simulink model "SelfAndRegularCheckouts"  (R2020a)
settings: Solver=VariableStepAuto  StartTime=0.0  StopTime=10.0  RelTol=1e-3
undefined symbols (not defined in the file): m, n
libraries: dspstat3 x1
settings Model: Creator=jggam  LastModifiedBy=jggam

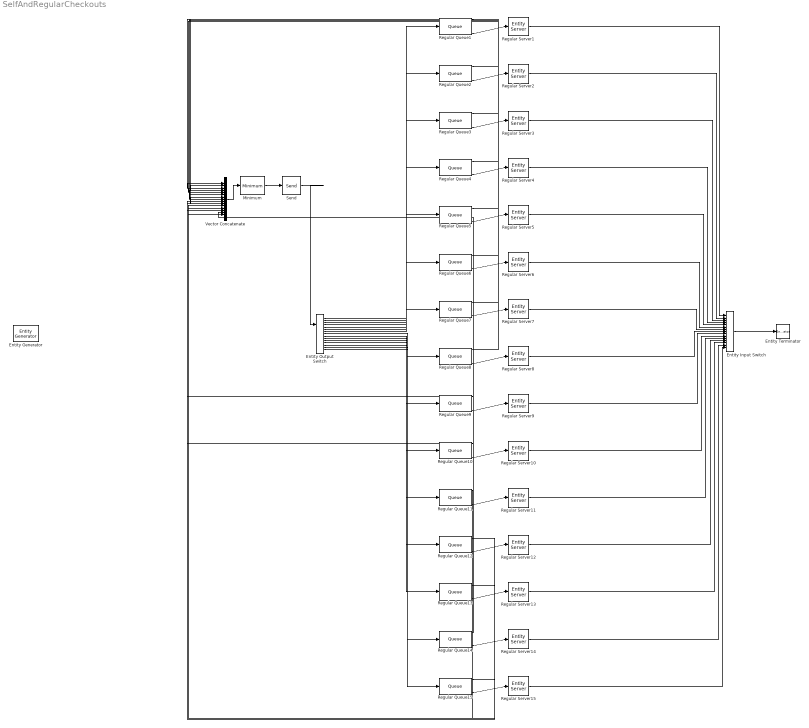
== system SelfAndRegularCheckouts ==
  Entity Input Switch : EntityInputSwitch  InputPortMessageModes=m,m,m,m,m,m,m,m,m,m,m,m,m,m,m  OutputPortMessageModes=m  NumberInputPorts=15
      settings: InputPortMap=u1,u2,u3,u4,u5,u6,u7,u8,u9,u10,u11,u12,u13,u14,u15
  Entity Output Switch : EntityOutputSwitch  InputPortMessageModes=m,m  OutputPortMessageModes=m,m,m,m,m,m,m,m,m,m,m,m,m,m,m  NumberOutputPorts=15  SwitchingCriterion=From control port  SwitchAttributeName=Attribute1
      settings: InputPortMap=u0,u1  OutputPortMap=o0,o1,o2,o3,o4,o5,o6,o7,o8,o9,o10,o11,o12,o13,o14
  Entity Generator : EntityGenerator  OutputPortMessageModes=n,m  TimeSource=MATLAB action  Period=0.5  IntergenerationTimeAction=dt = arrivalTime(RandArrivalTimesDist);  GenerateEntityAtSimulationStart=off  GenerateAction=|  AttributeName=NumberOfItems|ExpressEligible|RandomChoice  AttributeInitialValue=1|1|1  NumberEntitiesDeparted=on  EntityType=Structured  EntityTypeName=Entity
      | entity.NumberOfItems = numberOfItems(RandItemsDist);
      | if random() < 0.3
      |     entity.RandomChoice = 2;
      | else
      |     entity.RandomChoice = 1;
      | end
      settings: OutputPortMap=o0,o3
  Entity Terminator : EntityTerminator  InputPortMessageModes=m  NumberEntitiesArrived=on
      settings: OutputPortMap=o0
  Minimum : dspstat3/Minimum  operation=minimum  fcn=Index  indexBase=One  operateOver=Entire input  Dimension=1  InputProcessing=Columns as channels (frame based)  reset=None  roiEnable=off  roiType=Rectangles  roiPortion=Entire ROI  roiOutput=Individual statistics for each ROI  roiFlag=off  roundingMode=Floor  overflowMode=off
      settings: SourceProductBaseCode=DS
  Regular Queue{1..15} (15 alike) : Queue  InputPortMessageModes=m  OutputPortMessageModes=n,n,n,m  Capacity=RegularQueueCapacity  NumberEntitiesInBlock=on  AverageWait=on  AverageQueueLength=on
      settings: OutputPortMap=o1,o2,o3,o5
  Regular Server{1..15} (15 alike) : EntityServer  InputPortMessageModes=m  OutputPortMessageModes=m  Capacity=1  ServiceTimeSource=MATLAB action  ServiceTimeValue=1.75  ServiceTimeAction=dt = regularServiceTime(RandRegularServiceTimesDist);
  Send : Send  OutputPortMessageModes=m
  Vector Concatenate : Concatenate  NumInputs=15
  wires:
  Entity Output Switch/12 -> Regular Queue12/1
  Regular Queue14/4 -> Regular Server14/1
  Entity Output Switch/7 -> Regular Queue7/1
  Regular Queue4/4 -> Regular Server4/1
  Regular Server5/1 -> Entity Input Switch/5
  Entity Output Switch/10 -> Regular Queue10/1
  Regular Queue12/4 -> Regular Server12/1
  Regular Queue11/4 -> Regular Server11/1
  Regular Queue8/1 -> Vector Concatenate/8
  Regular Server10/1 -> Entity Input Switch/10
  Regular Queue13/1 -> Vector Concatenate/13
  Regular Queue5/1 -> Vector Concatenate/5
  Regular Queue4/1 -> Vector Concatenate/4
  Regular Server3/1 -> Entity Input Switch/3
  Regular Server4/1 -> Entity Input Switch/4
  Regular Server6/1 -> Entity Input Switch/6
  Minimum/1 -> Send/1
  Regular Server1/1 -> Entity Input Switch/1
  Regular Queue13/4 -> Regular Server13/1
  Regular Queue1/1 -> Vector Concatenate/1
  Regular Server7/1 -> Entity Input Switch/7
  Regular Queue5/4 -> Regular Server5/1
  Regular Queue14/1 -> Vector Concatenate/14
  Entity Output Switch/8 -> Regular Queue8/1
  Regular Queue8/4 -> Regular Server8/1
  Regular Queue2/1 -> Vector Concatenate/2
  Regular Server15/1 -> Entity Input Switch/15
  Regular Server13/1 -> Entity Input Switch/13
  Vector Concatenate/1 -> Minimum/1
  Regular Server8/1 -> Entity Input Switch/8
  Regular Queue7/1 -> Vector Concatenate/7
  Regular Server12/1 -> Entity Input Switch/12
  Regular Server11/1 -> Entity Input Switch/11
  Entity Output Switch/5 -> Regular Queue5/1
  Entity Output Switch/2 -> Regular Queue2/1
  Regular Queue3/4 -> Regular Server3/1
  Regular Queue6/4 -> Regular Server6/1
  Regular Queue2/4 -> Regular Server2/1
  Regular Queue3/1 -> Vector Concatenate/3
  Entity Output Switch/4 -> Regular Queue4/1
  Entity Input Switch/1 -> Entity Terminator/1
  Entity Output Switch/9 -> Regular Queue9/1
  Entity Output Switch/11 -> Regular Queue11/1
  Regular Queue15/4 -> Regular Server15/1
  Entity Output Switch/13 -> Regular Queue13/1
  Entity Output Switch/6 -> Regular Queue6/1
  Entity Output Switch/14 -> Regular Queue14/1
  Send/1 -> Entity Output Switch/1
  Regular Queue9/1 -> Vector Concatenate/9
  Entity Output Switch/3 -> Regular Queue3/1
  Regular Queue7/4 -> Regular Server7/1
  Regular Queue15/1 -> Vector Concatenate/15
  Regular Queue9/4 -> Regular Server9/1
  Regular Queue10/1 -> Vector Concatenate/10
  Entity Output Switch/1 -> Regular Queue1/1
  Regular Server14/1 -> Entity Input Switch/14
  Regular Server9/1 -> Entity Input Switch/9
  Regular Server2/1 -> Entity Input Switch/2
  Regular Queue11/1 -> Vector Concatenate/11
  Regular Queue1/4 -> Regular Server1/1
  Regular Queue6/1 -> Vector Concatenate/6
  Regular Queue10/4 -> Regular Server10/1
  Regular Queue12/1 -> Vector Concatenate/12
  Entity Output Switch/15 -> Regular Queue15/1
